simulink model "Joystick_check"  (R2014a)
settings: Solver=ode45  StartTime=0.0  StopTime=inf  RelTol=1e-3
libraries: vrlib x1, realtime_pacer_lib x1
settings Model: Creator=p-narayan  LastModifiedBy=p-narayan

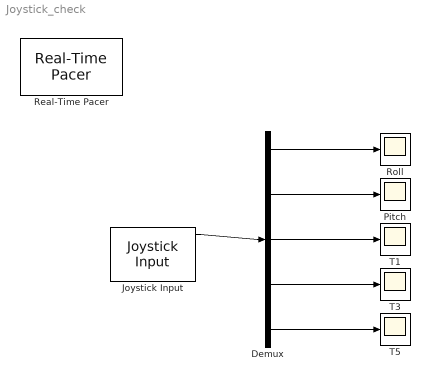
== system Joystick_check ==
  Demux : Demux  Outputs=5
  Joystick Input : vrlib/Joystick Input  joyid=1  adjustports=on  forcefeed=off
  Pitch : Scope
  Real-Time Pacer : realtime_pacer_lib/Real-Time Pacer  simTimePerRealTime=1
  Roll : Scope
      settings: SaveName=ScopeData2
  T1 : Scope
  T3 : Scope
      settings: SaveName=ScopeData3
  T5 : Scope
      settings: SaveName=ScopeData4
  wires:
  Demux/1 -> Roll/1
  Demux/2 -> Pitch/1
  Demux/3 -> T1/1
  Demux/4 -> T3/1
  Demux/5 -> T5/1
  Joystick Input/1 -> Demux/1
